simulink model "lab2_3"  (R2023a)
settings: Solver=VariableStepAuto  StartTime=0.0  StopTime=10.0  RelTol=1e-3
undefined symbols (not defined in the file or in its folder): C, K, Le, x0
settings Model: Creator=bz  LastModifiedBy=bz

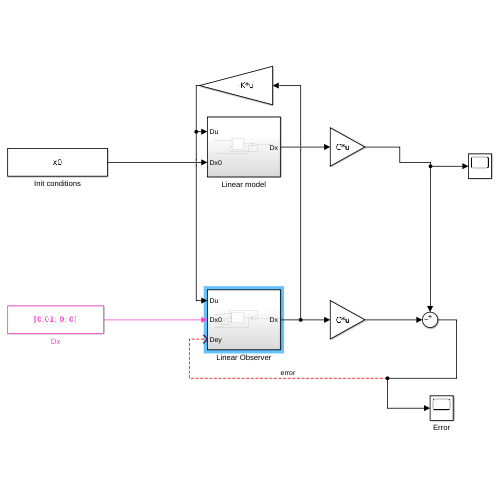
[thumbnail: Simulink's stored preview of the top-level diagram]
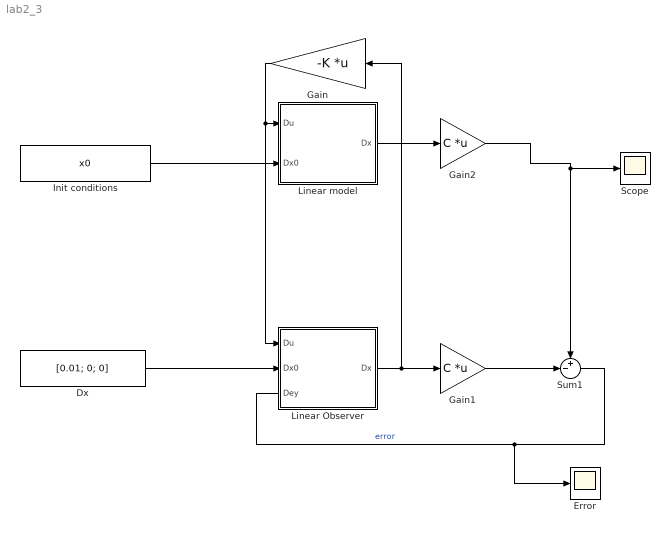
== system lab2_3 ==
  Dx : Constant  Value=[0.01; 0; 0]  VectorParams1D=off
  Error : Scope
  Gain : Gain  Gain=-K  Multiplication=Matrix(K*u)
  Gain1 : Gain  Gain=C  Multiplication=Matrix(K*u)
  Gain2 : Gain  Gain=C  Multiplication=Matrix(K*u)
  Init conditions : Constant  Value=x0  VectorParams1D=off
  Linear Observer : Subsystem
  Linear model : Subsystem
  Scope : Scope
  Sum1 : Sum  Inputs=+-|
  wires:
  Gain/1 -> Linear Observer/1(Du), Linear model/1(Du)
  Init conditions/1 -> Linear model/2(Dx0)
  Dx/1 -> Linear Observer/2(Dx0)
  Linear Observer/1(Dx) -> Gain/1, Gain1/1
  Gain1/1 -> Sum1/2
  Linear model/1(Dx) -> Gain2/1
  Gain2/1 -> Scope/1, Sum1/1
  Sum1/1 -> Error/1  "error"

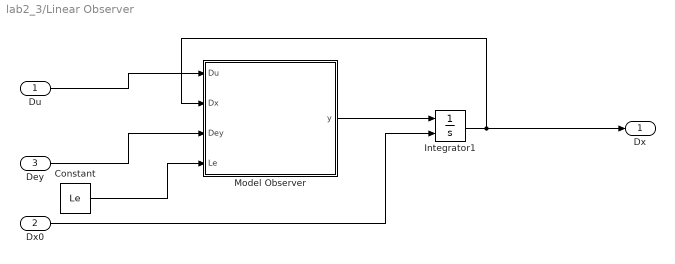
== system lab2_3/Linear Observer ==
  Du : Inport
  Dx0 : Inport  Port=2
  Dey : Inport  Port=3
  Constant : Constant  Value=Le
  Integrator1 : Integrator  InitialConditionSource=external
  Model Observer : MATLAB Function  TreatAsAtomicUnit=on
  Dx : Outport
  wires:
  Model Observer/1(y) -> Integrator1/1
  Dx0/1 -> Integrator1/2
  Integrator1/1 -> Dx/1, Model Observer/2(Dx)
  Du/1 -> Model Observer/1(Du)
  Dey/1 -> Model Observer/3(Dey)
  Constant/1 -> Model Observer/4(Le)

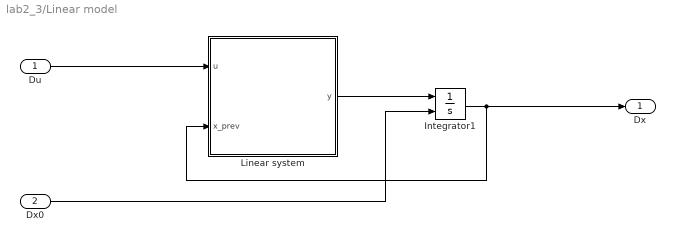
== system lab2_3/Linear model ==
  Du : Inport
  Dx0 : Inport  Port=2
  Integrator1 : Integrator  InitialConditionSource=external
  Linear system : MATLAB Function  TreatAsAtomicUnit=on
  Dx : Outport
  wires:
  Linear system/1(y) -> Integrator1/1
  Dx0/1 -> Integrator1/2
  Integrator1/1 -> Dx/1, Linear system/2(x_prev)
  Du/1 -> Linear system/1(u)

== matlab function lab2_3/Linear model/Linear system ==
  data: u input; y output size=[3,1]; x_prev input
function y  = fcn(u, x_prev)

A = [0              0.0010      0;
     1.6847         0           -0.0257;
     0              0           -0.2888] * 1e3;

B = [0;
     0;
     1.2706] * 1e3;

y = A * x_prev + B * u;

end

== matlab function lab2_3/Linear Observer/Model Observer ==
  data: Du input; y output size=[3,1]; Dx input; Dey input; Le input
function y  = observer(Du, Dx, Dey, Le)

A = [0              0.0010      0;
     1.6847         0           -0.0257;
     0              0           -0.2888] * 1e3;

E = [1; 0; 0];

Ae = [A E;
     zeros(1, 4)];

B = [0;
     0;
     1.2706] * 1e3;

Be = [B; 0];

y = Ae * Dx + Be * Du + Le * Dey;

end
